simulink model "Lab_1_part_2"  (R2019b)
settings: Solver=VariableStepAuto  StartTime=0.0  StopTime=10.0  RelTol=1e-3
libraries: dspstat3 x3, dspmathops x3, dsparch4 x2, dspsrcs4 x1, simulink x1, powerlib_meascontrol x1
settings Model: Creator=qiuzh  LastModifiedBy=mikewang
settings DataIOCC: ReturnWorkspaceOutputs=off
settings DebuggingCC: ArithmeticOperatorsInVariantConditions=warning
settings SFSimCC: SimUseLocalCustomCode=off  CustomCodeUndefinedFunction=UseInterfaceOnly
settings RTWCC: RTWUseLocalCustomCode=off

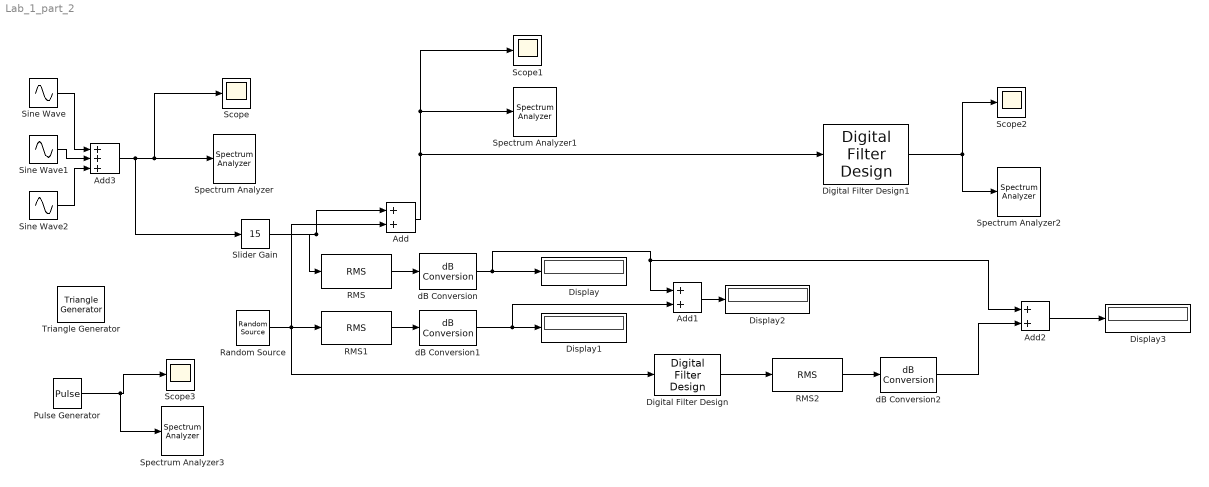
== system Lab_1_part_2 ==
  Add : Sum
  Add1 : Sum
  Add2 : Sum
  Add3 : Sum  Inputs=+++
  Digital Filter Design : dsparch4/Digital Filter Design  mwdsp_browser_bugfix_var=off
  Digital Filter Design1 : dsparch4/Digital Filter Design  mwdsp_browser_bugfix_var=off
  Display{,1..3} (4 alike) : Display
  Pulse Generator : DiscretePulseGenerator  Period=100  PulseWidth=50  SampleTime=1e-6
  RMS : dspstat3/RMS  run=on  directionMode=Each column  dimension=1  InputProcessing=Columns as channels (frame based)  reset_popup=None
  RMS1 : dspstat3/RMS  run=off  directionMode=Each column  dimension=1  InputProcessing=Columns as channels (frame based)  reset_popup=None
  RMS2 : dspstat3/RMS  run=on  directionMode=Each column  dimension=1  InputProcessing=Columns as channels (frame based)  reset_popup=None
  Random Source : dspsrcs4/Random Source  SrcType=Gaussian  NormMethod=Ziggurat  CltLength=12  MinVal=0  MaxVal=1  MeanVal=0  VarVal=1  RepMode=Not repeatable  rawSeed=1  IsInherit=off  SampMode=Discrete  SampTime=1e-6  SampFrame=1  DataType=Double  OutComplex=Real  OutputFrames=off
  Scope{,1..3} (4 alike) : Scope
  Sine Wave : Sin  SineType=Sample based  Samples=100  SampleTime=1e-6
  Sine Wave1 : Sin  SineType=Sample based  Samples=50  SampleTime=1e-6
  Sine Wave2 : Sin  SineType=Sample based  Samples=200  SampleTime=1e-6
  Slider Gain : simulink/Math Operations/Slider Gain  gain=15  low=0  high=20
  Spectrum Analyzer{,1..3} (4 alike) : SpectrumAnalyzer
  Triangle Generator : powerlib_meascontrol/Pulse & Signal Generators/Triangle Generator  Freq=1e4  Phase=90  Ts=1e-6
      settings: SourceProductName=Simscape Electrical
  dB Conversion : dspmathops/dB Conversion  dBtype=dB  intype=Amplitude  R=1  fuzz=off
      settings: SourceProductName=DSP System Toolbox
  dB Conversion1 : dspmathops/dB Conversion  dBtype=dB  intype=Amplitude  R=1  fuzz=off
      settings: SourceProductName=DSP System Toolbox
  dB Conversion2 : dspmathops/dB Conversion  dBtype=dB  intype=Amplitude  R=1  fuzz=off
      settings: SourceProductName=DSP System Toolbox
  wires:
  Slider Gain/1 -> Add/1, RMS/1
  RMS1/1 -> dB Conversion1/1
  Random Source/1 -> Digital Filter Design/1, Add/2, RMS1/1
  dB Conversion1/1 -> Add1/2, Display1/1
  Add/1 -> Scope1/1, Spectrum Analyzer1/1, Digital Filter Design1/1
  dB Conversion/1 -> Add1/1, Add2/1, Display/1
  RMS/1 -> dB Conversion/1
  Digital Filter Design1/1 -> Spectrum Analyzer2/1, Scope2/1
  Add1/1 -> Display2/1
  RMS2/1 -> dB Conversion2/1
  Digital Filter Design/1 -> RMS2/1
  dB Conversion2/1 -> Add2/2
  Add2/1 -> Display3/1
  Pulse Generator/1 -> Scope3/1, Spectrum Analyzer3/1
  Sine Wave/1 -> Add3/1
  Sine Wave1/1 -> Add3/2
  Sine Wave2/1 -> Add3/3
  Add3/1 -> Slider Gain/1, Scope/1, Spectrum Analyzer/1
